simulink model "BCD"  (R2025a)
settings: Solver=FixedStepDiscrete  StartTime=0.0  StopTime=10  MaxStep=0.2  RelTol=1e-3
libraries: simulink x14
settings Model: Creator=HomePC  LastModifiedBy=HomePC

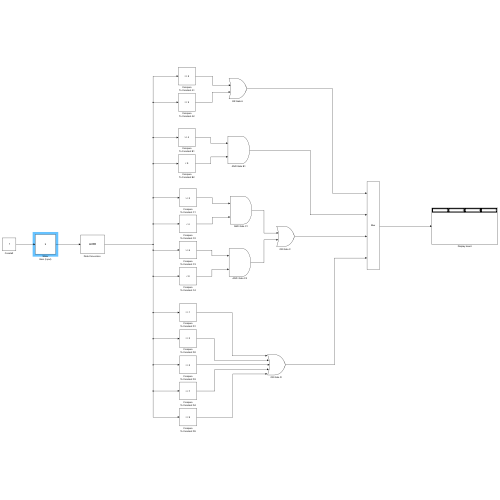
[thumbnail: Simulink's stored preview of the top-level diagram]
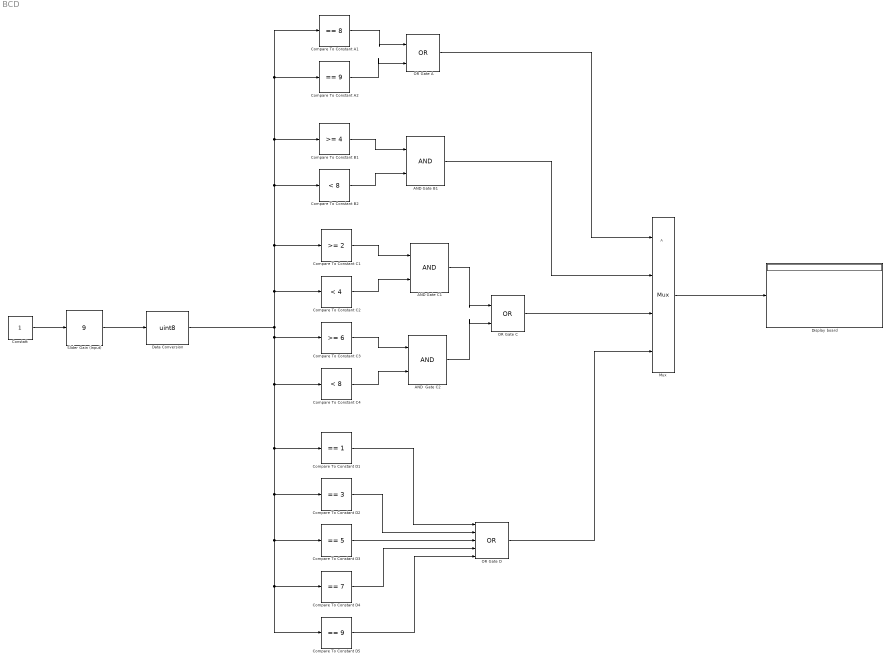
== system BCD ==
  note: A
  AND  Gate C2 : Logic  IconShape=distinctive  AllPortsSameDT=off  OutDataTypeStr=boolean
  AND Gate B1 : Logic  IconShape=distinctive  AllPortsSameDT=off  OutDataTypeStr=boolean
  AND Gate C1 : Logic  IconShape=distinctive  AllPortsSameDT=off  OutDataTypeStr=boolean
  Compare To Constant A1 : simulink/Logic and Bit Operations/Compare To Constant  relop===  const=8  OutDataTypeStr=boolean
  Compare To Constant A2 : simulink/Logic and Bit Operations/Compare To Constant  relop===  const=9  OutDataTypeStr=boolean
  Compare To Constant B1 : simulink/Logic and Bit Operations/Compare To Constant  relop=>=  const=4  OutDataTypeStr=boolean
  Compare To Constant B2 : simulink/Logic and Bit Operations/Compare To Constant  relop=<  const=8  OutDataTypeStr=boolean
  Compare To Constant C1 : simulink/Logic and Bit Operations/Compare To Constant  relop=>=  const=2  OutDataTypeStr=boolean
  Compare To Constant C2 : simulink/Logic and Bit Operations/Compare To Constant  relop=<  const=4  OutDataTypeStr=boolean
  Compare To Constant C3 : simulink/Logic and Bit Operations/Compare To Constant  relop=>=  const=6  OutDataTypeStr=boolean
  Compare To Constant C4 : simulink/Logic and Bit Operations/Compare To Constant  relop=<  const=8  OutDataTypeStr=boolean
  Compare To Constant D1 : simulink/Logic and Bit Operations/Compare To Constant  relop===  const=1  OutDataTypeStr=boolean
  Compare To Constant D2 : simulink/Logic and Bit Operations/Compare To Constant  relop===  const=3  OutDataTypeStr=boolean
  Compare To Constant D3 : simulink/Logic and Bit Operations/Compare To Constant  relop===  const=5  OutDataTypeStr=boolean
  Compare To Constant D4 : simulink/Logic and Bit Operations/Compare To Constant  relop===  const=7  OutDataTypeStr=boolean
  Compare To Constant D5 : simulink/Logic and Bit Operations/Compare To Constant  relop===  const=9  OutDataTypeStr=boolean
  Constatt : Constant
  "Data Conversion " : DataTypeConversion  OutDataTypeStr=uint8  SaturateOnIntegerOverflow=off  RndMeth=Floor
  Display board : Display
  Mux : Mux
  OR Gate A : Logic  Operator=OR  IconShape=distinctive  AllPortsSameDT=off  OutDataTypeStr=boolean
  OR Gate C : Logic  Operator=OR  IconShape=distinctive  AllPortsSameDT=off  OutDataTypeStr=boolean
  OR Gate D : Logic  Operator=OR  Inputs=5  IconShape=distinctive  AllPortsSameDT=off  OutDataTypeStr=boolean
  Slider Gain (Input) : simulink/Math Operations/Slider Gain  gain=9  low=0  high=9
  wires:
  Compare To Constant B1/1 -> AND Gate B1/1
  Compare To Constant B2/1 -> AND Gate B1/2
  Compare To Constant C1/1 -> AND Gate C1/1
  Compare To Constant C2/1 -> AND Gate C1/2
  Compare To Constant C3/1 -> AND  Gate C2/1
  Compare To Constant C4/1 -> AND  Gate C2/2
  AND Gate C1/1 -> OR Gate C/1
  AND  Gate C2/1 -> OR Gate C/2
  OR Gate C/1 -> Mux/3
  AND Gate B1/1 -> Mux/2
  OR Gate D/1 -> Mux/4
  Mux/1 -> Display board/1
  "Data Conversion "/1 -> Compare To Constant A1/1, Compare To Constant A2/1, Compare To Constant B1/1, Compare To Constant B2/1, Compare To Constant C1/1, Compare To Constant C2/1, Compare To Constant D2/1, Compare To Constant D3/1, Compare To Constant D5/1, Compare To Constant D4/1, Compare To Constant D1/1, Compare To Constant C4/1, Compare To Constant C3/1
  Compare To Constant D3/1 -> OR Gate D/3
  Compare To Constant D1/1 -> OR Gate D/1
  Compare To Constant D2/1 -> OR Gate D/2
  Compare To Constant D4/1 -> OR Gate D/4
  Compare To Constant D5/1 -> OR Gate D/5
  Compare To Constant A1/1 -> OR Gate A/1
  Compare To Constant A2/1 -> OR Gate A/2
  OR Gate A/1 -> Mux/1
  Slider Gain (Input)/1 -> "Data Conversion "/1
  Constatt/1 -> Slider Gain (Input)/1
